simulink model "test_fmu"  (R2022a)
settings: Solver=FixedStepAuto  StartTime=0.0  StopTime=10.0  RelTol=1e-3
settings Model: Creator=lordx  LastModifiedBy=lordx
settings OptimizationCC: UseDivisionForNetSlopeComputation=on  OptimizeBlockIOStorage=off  InitFltsAndDblsToZero=on  EfficientMapNaN2IntZero=off  BufferReusableBoundary=off
settings HardwareCC: TargetBitPerPointer=64  TargetBitPerSizeT=64  TargetBitPerPtrDiffT=64  TargetLongLongMode=on  TargetIntDivRoundTo=Zero  TargetEndianess=LittleEndian  TargetWordSize=64  TargetHWDeviceType=MATLAB Host  ProdEqTarget=off
settings RTWCC: Description=FMU based on GRT (Functional Mock-up Unit)  SystemTargetFile=grtfmi.tlc  GenerateMakefile=off  TemplateMakefile=none  GenerateReport=on  RetainRTWFile=on
settings CodeAppCC: ForceParamTrailComments=on  StateflowObjectComments=on  MATLABSourceComments=on
settings STFCustomTargetCC: TargetLangStandard=C99 (ISO)  CombineOutputUpdateFcns=on  GRTInterface=off  SystemTargetFile=grtfmi.tlc
settings GRTTargetCC: ParMdlRefBuildCompliant=off  CompOptLevelCompliant=off  ConcurrentExecutionCompliant=off  MatFileLogging=off  CPPClassGenCompliant=off  UseToolchainInfoCompliant=off  RTWCAPISignals=on  RTWCAPIParams=on  RTWCAPIStates=on  RTWCAPIRootIO=on

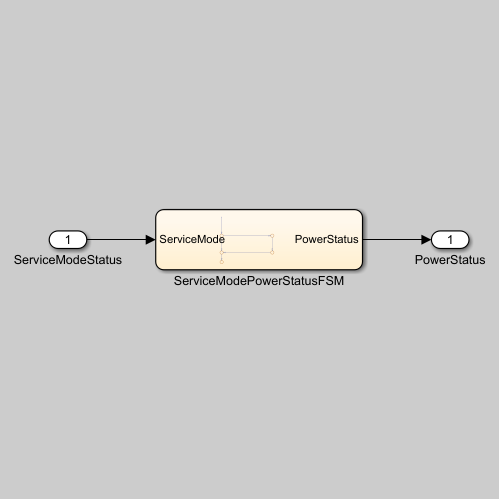
[thumbnail: Simulink's stored preview of the top-level diagram]
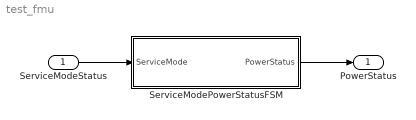
== system test_fmu ==
  ServiceModeStatus : Inport
  ServiceModePowerStatusFSM : Stateflow chart  TreatAsAtomicUnit=on
  PowerStatus : Outport
  wires:
  ServiceModeStatus/1 -> ServiceModePowerStatusFSM/1(ServiceMode)
  ServiceModePowerStatusFSM/1(PowerStatus) -> PowerStatus/1

== stateflow chart test_fmu/ServiceModePowerStatusFSM ==
  (default) -> (junction 8) : /* Service Mode State Machine */
  (junction 8) -> (junction 4) [order 1] : [ServiceMode != 0]
  (junction 8) -> (junction 1) [order 2] : {PowerStatus = 0;}
  (junction 4) -> (junction 9) : {PowerStatus = 1;}
  (junction 9) -> (junction 1) : [ServiceMode == 0]
  (junction 1) -> (junction 6)
  data: ServiceMode input; PowerStatus output double
